simulink model "Level3Model"  (R2023b)
settings: Solver=VariableStepAuto  StartTime=0.0  StopTime=5  FixedStep=0.01  RelTol=1e-3
undefined symbols (not defined in the file or in its folder): A, B, C, Ke, Kr, uD
settings Model: Creator=abane  LastModifiedBy=vikhy
settings OptimizationCC: ReuseModelBlockBuffer=off

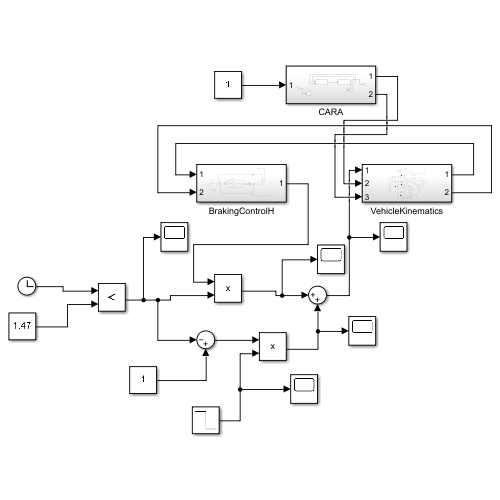
[thumbnail: Simulink's stored preview of the top-level diagram]
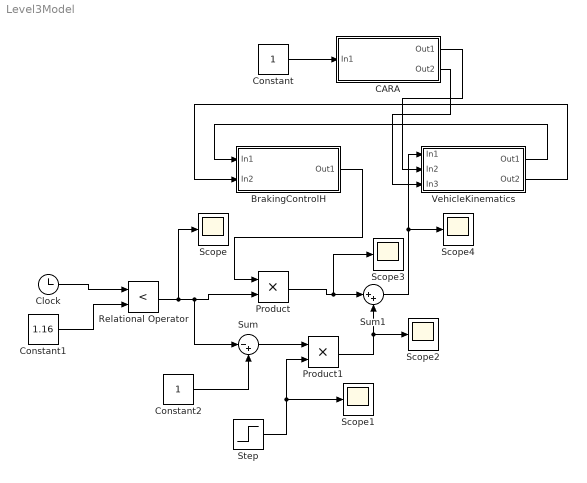
== system Level3Model ==
  BrakingControlH : Subsystem
  CARA : Subsystem
  Clock : Clock
  Constant : Constant
  Constant1 : Constant  Value=1.16
  Constant2 : Constant
  Product : Product
  Product1 : Product
  Relational Operator : RelationalOperator  Operator=<  OutDataTypeStr=boolean  RndMeth=Simplest  InputSameDT=off
  Scope{,1..4} (5 alike) : Scope
  Step : Step  Time=1.16  After=-220  SampleTime=0
  Sum : Sum  Inputs=|-+
  Sum1 : Sum  Inputs=|++
  VehicleKinematics : Subsystem
  wires:
  VehicleKinematics/1(Out1) -> BrakingControlH/1(In1)
  VehicleKinematics/2(Out2) -> BrakingControlH/2(In2)
  Constant/1 -> CARA/1(In1)
  CARA/1(Out1) -> VehicleKinematics/2(In2)
  CARA/2(Out2) -> VehicleKinematics/3(In3)
  Clock/1 -> Relational Operator/1
  Constant1/1 -> Relational Operator/2
  BrakingControlH/1(Out1) -> Product/1
  Relational Operator/1 -> Scope/1, Sum/1, Product/2
  Constant2/1 -> Sum/2
  Sum/1 -> Product1/1
  Step/1 -> Scope1/1, Product1/2
  Product/1 -> Scope3/1, Sum1/1
  Product1/1 -> Scope2/1, Sum1/2
  Sum1/1 -> VehicleKinematics/1(In1), Scope4/1

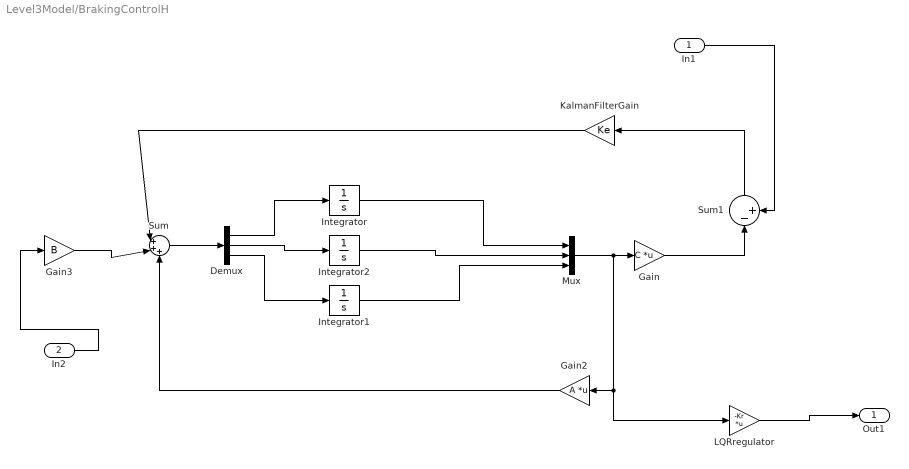
== system Level3Model/BrakingControlH ==
  In1 : Inport
  In2 : Inport  Port=2
  Demux : Demux  Outputs=3
  Gain : Gain  Gain=C  Multiplication=Matrix(K*u)
  Gain2 : Gain  Gain=A  Multiplication=Matrix(K*u)
  Gain3 : Gain  Gain=B
  Integrator : Integrator
  Integrator1 : Integrator
  Integrator2 : Integrator
  KalmanFilterGain : Gain  Gain=Ke
  LQRregulator : Gain  Gain=-Kr  Multiplication=Matrix(K*u)
  Mux : Mux  Inputs=3
  Sum : Sum  Inputs=|+++
  Sum1 : Sum  Inputs=|-+
  Out1 : Outport
  wires:
  Sum/1 -> Demux/1
  Demux/1 -> Integrator/1
  Demux/3 -> Integrator1/1
  Integrator/1 -> Mux/1
  Integrator1/1 -> Mux/3
  Mux/1 -> LQRregulator/1, Gain2/1, Gain/1
  Gain/1 -> Sum1/1
  Sum1/1 -> KalmanFilterGain/1
  KalmanFilterGain/1 -> Sum/1
  Gain2/1 -> Sum/3
  Gain3/1 -> Sum/2
  LQRregulator/1 -> Out1/1
  In2/1 -> Gain3/1
  Demux/2 -> Integrator2/1
  Integrator2/1 -> Mux/2
  In1/1 -> Sum1/2

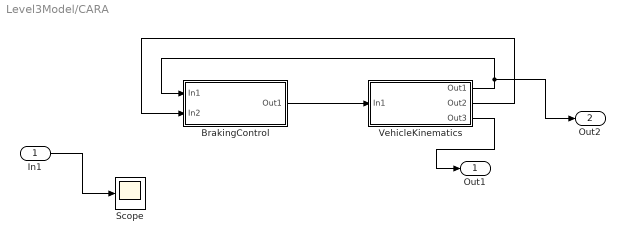
== system Level3Model/CARA ==
  In1 : Inport
  BrakingControl : Subsystem
  Scope : Scope
  VehicleKinematics : Subsystem
  Out1 : Outport
  Out2 : Outport  Port=2
  wires:
  VehicleKinematics/2(Out2) -> BrakingControl/2(In2)
  VehicleKinematics/1(Out1) -> Out2/1, BrakingControl/1(In1)
  BrakingControl/1(Out1) -> VehicleKinematics/1(In1)
  VehicleKinematics/3(Out3) -> Out1/1
  In1/1 -> Scope/1

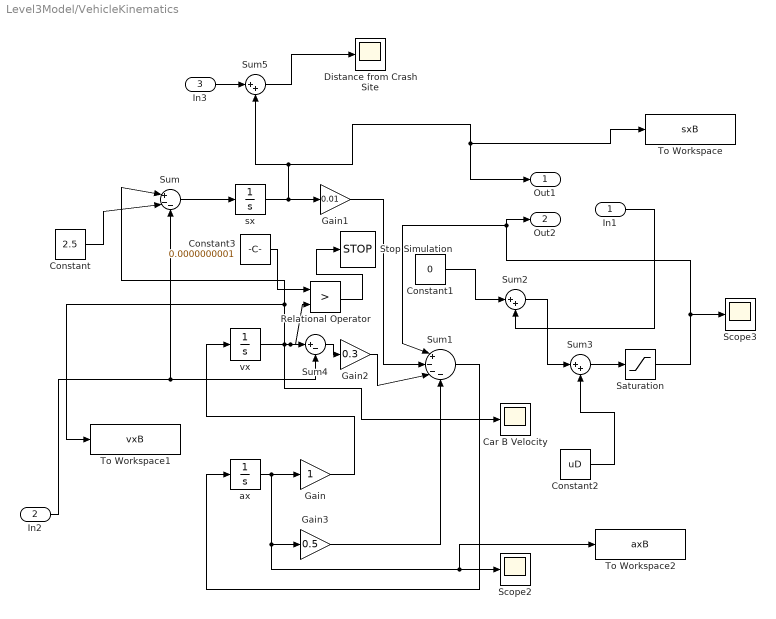
== system Level3Model/VehicleKinematics ==
  In1 : Inport
  In2 : Inport  Port=2
  In3 : Inport  Port=3
  Car B Velocity : Scope
  Constant : Constant  Value=2.5
  Constant1 : Constant  Value=0
  Constant2 : Constant  Value=uD
  Constant3 : Constant  Value=0.0000000001
  Distance from Crash Site : Scope
  Gain : Gain
  Gain1 : Gain  Gain=0.01
  Gain2 : Gain  Gain=0.3
  Gain3 : Gain  Gain=0.5
  Relational Operator : RelationalOperator  Operator=>  OutDataTypeStr=boolean  RndMeth=Simplest  InputSameDT=off
  Saturation : Saturate  UpperLimit=0  LowerLimit=-20000
  Scope2 : Scope
  Scope3 : Scope
  Stop Simulation : Stop
  Sum : Sum  Inputs=|+--
  Sum1 : Sum  Inputs=|+---
  Sum2 : Sum  Inputs=|++
  Sum3 : Sum  Inputs=|++
  Sum4 : Sum  Inputs=|+-
  Sum5 : Sum  Inputs=|++
  To Workspace : ToWorkspace  VariableName=sxB  SaveFormat=Timeseries  SampleTime=-1
  To Workspace1 : ToWorkspace  VariableName=vxB  SaveFormat=Timeseries  SampleTime=-1
  To Workspace2 : ToWorkspace  VariableName=axB  SaveFormat=Timeseries  SampleTime=-1
  ax : Integrator
  sx : Integrator  InitialCondition=-43.8
  vx : Integrator  InitialCondition=60
  Out1 : Outport
  Out2 : Outport  Port=2
  wires:
  Constant/1 -> Sum/2
  Sum3/1 -> Saturation/1
  Constant2/1 -> Sum3/2
  Gain1/1 -> Sum1/2
  vx/1 -> Car B Velocity/1, To Workspace1/1, Sum/1, Relational Operator/2, Sum4/1
  Saturation/1 -> Out2/1, Sum1/1, Scope3/1
  Gain3/1 -> Sum1/4
  Sum1/1 -> ax/1
  sx/1 -> Out1/1, To Workspace/1, Sum5/2, Gain1/1
  Sum2/1 -> Sum3/1
  ax/1 -> To Workspace2/1, Scope2/1, Gain3/1, Gain/1
  In1/1 -> Sum2/2
  Gain2/1 -> Sum1/3
  Constant1/1 -> Sum2/1
  Gain/1 -> vx/1
  Sum/1 -> sx/1
  Relational Operator/1 -> Stop Simulation/1
  Constant3/1 -> Relational Operator/1
  In2/1 -> Sum/3, Sum4/2
  Sum4/1 -> Gain2/1
  In3/1 -> Sum5/1
  Sum5/1 -> Distance from Crash Site/1

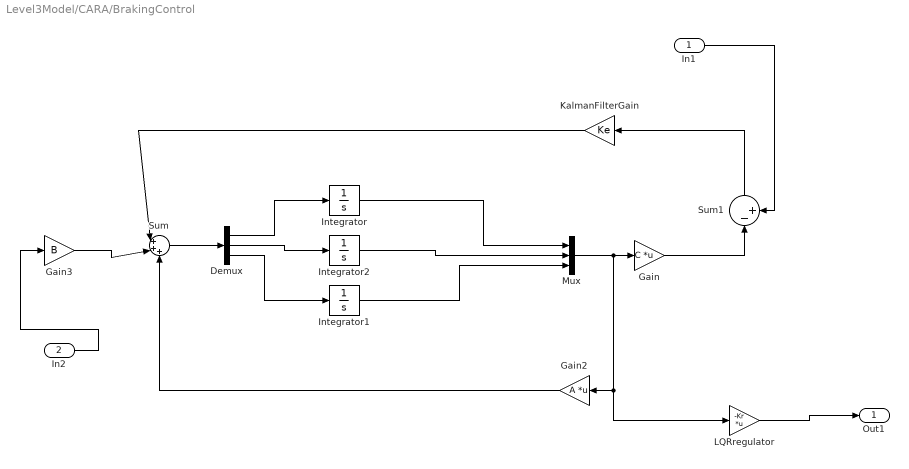
== system Level3Model/CARA/BrakingControl ==
  In1 : Inport
  In2 : Inport  Port=2
  Demux : Demux  Outputs=3
  Gain : Gain  Gain=C  Multiplication=Matrix(K*u)
  Gain2 : Gain  Gain=A  Multiplication=Matrix(K*u)
  Gain3 : Gain  Gain=B
  Integrator : Integrator
  Integrator1 : Integrator
  Integrator2 : Integrator
  KalmanFilterGain : Gain  Gain=Ke
  LQRregulator : Gain  Gain=-Kr  Multiplication=Matrix(K*u)
  Mux : Mux  Inputs=3
  Sum : Sum  Inputs=|+++
  Sum1 : Sum  Inputs=|-+
  Out1 : Outport
  wires:
  Sum/1 -> Demux/1
  Demux/1 -> Integrator/1
  Demux/3 -> Integrator1/1
  Integrator/1 -> Mux/1
  Integrator1/1 -> Mux/3
  Mux/1 -> LQRregulator/1, Gain2/1, Gain/1
  Gain/1 -> Sum1/1
  Sum1/1 -> KalmanFilterGain/1
  KalmanFilterGain/1 -> Sum/1
  Gain2/1 -> Sum/3
  Gain3/1 -> Sum/2
  LQRregulator/1 -> Out1/1
  In2/1 -> Gain3/1
  Demux/2 -> Integrator2/1
  Integrator2/1 -> Mux/2
  In1/1 -> Sum1/2

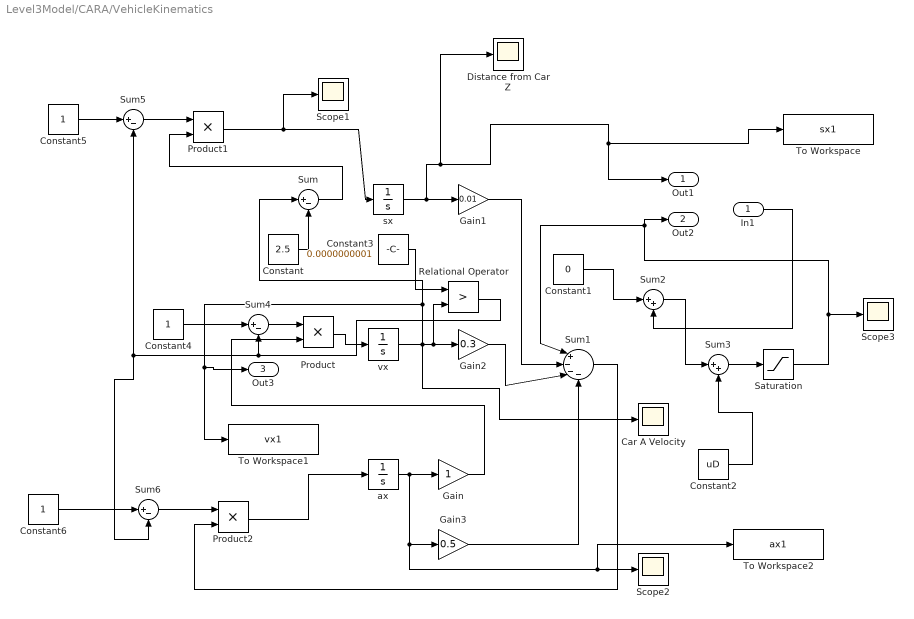
== system Level3Model/CARA/VehicleKinematics ==
  In1 : Inport
  Car A Velocity : Scope
  Constant : Constant  Value=2.5
  Constant1 : Constant  Value=0
  Constant2 : Constant  Value=uD
  Constant3 : Constant  Value=0.0000000001
  Constant4 : Constant
  Constant5 : Constant
  Constant6 : Constant
  Distance from Car Z : Scope
  Gain : Gain
  Gain1 : Gain  Gain=0.01
  Gain2 : Gain  Gain=0.3
  Gain3 : Gain  Gain=0.5
  Product : Product
  Product1 : Product
  Product2 : Product
  Relational Operator : RelationalOperator  Operator=>  OutDataTypeStr=boolean  RndMeth=Simplest  InputSameDT=off
  Saturation : Saturate  UpperLimit=0  LowerLimit=-200
  Scope1 : Scope
  Scope2 : Scope
  Scope3 : Scope
  Sum{,4..6} (4 alike) : Sum  Inputs=|+-
  Sum1 : Sum  Inputs=|+---
  Sum2 : Sum  Inputs=|++
  Sum3 : Sum  Inputs=|++
  To Workspace : ToWorkspace  VariableName=sx1  SaveFormat=Timeseries  SampleTime=-1
  To Workspace1 : ToWorkspace  VariableName=vx1  SaveFormat=Timeseries  SampleTime=-1
  To Workspace2 : ToWorkspace  VariableName=ax1  SaveFormat=Timeseries  SampleTime=-1
  ax : Integrator
  sx : Integrator  InitialCondition=-43.8
  vx : Integrator  InitialCondition=35
  Out1 : Outport
  Out2 : Outport  Port=2
  Out3 : Outport  Port=3
  wires:
  Constant/1 -> Sum/2
  Sum3/1 -> Saturation/1
  Constant2/1 -> Sum3/2
  Gain1/1 -> Sum1/2
  vx/1 -> Car A Velocity/1, Out3/1, To Workspace1/1, Sum/1, Relational Operator/2, Gain2/1
  Saturation/1 -> Out2/1, Sum1/1, Scope3/1
  Gain3/1 -> Sum1/4
  Sum1/1 -> Product2/2
  sx/1 -> Distance from Car Z/1, Out1/1, To Workspace/1, Gain1/1
  Sum2/1 -> Sum3/1
  ax/1 -> To Workspace2/1, Scope2/1, Gain3/1, Gain/1
  In1/1 -> Sum2/2
  Gain2/1 -> Sum1/3
  Constant1/1 -> Sum2/1
  Constant3/1 -> Relational Operator/1
  Sum4/1 -> Product/1
  Relational Operator/1 -> Sum6/2, Sum5/2, Sum4/2
  Constant4/1 -> Sum4/1
  Gain/1 -> Product/2
  Product/1 -> vx/1
  Constant5/1 -> Sum5/1
  Sum5/1 -> Product1/1
  Sum/1 -> Product1/2
  Product1/1 -> Scope1/1, sx/1
  Constant6/1 -> Sum6/1
  Sum6/1 -> Product2/1
  Product2/1 -> ax/1
